simulink model "L4_MABX"  (R2018a)
settings: Solver=FixedStepDiscrete  StartTime=0.0  StopTime=Inf  FixedStep=0.01  RelTol=1e-3  EnableMultiTasking=on
PostLoadFcn:
  | , if any(exist('dsrtsu_mdlpostloadfcn', 'file') == [2, 3, 6]), try dsrtsu_mdlpostloadfcn('Execute', bdroot); catch fprintf('Error in PostLoadFcn (dsrtsu_mdlpostloadfcn) for model "%s":\n %s\n', bdroot, lasterr); end, end,
InitFcn:
  | disp([ptc_matlab_lib.isodatetime ' - ' bdroot(gcs) ' - Setting FixedStep to GLB_FIXED_STEP_SIZE_CPV']);
  | set_param(bdroot(gcs), 'FixedStep', num2str(GLB_FIXED_STEP_SIZE_CPV.Value));
undefined symbols (not defined in the file or in its folder): dsa_RTMapsManager, ENUM_CAN_STATUS_DIAG_T
libraries: PTC_MBDS_LIB x14, rtican x12, dsa_tcpip_lib x2, SUB_ECU_L4_MABX_HW_Interface_PIC_KW x2, rtiethxcplib x2, SUB_ECU_L4_MABX x1, simulink x1, rtmapslib x1
(part 2 of 2)

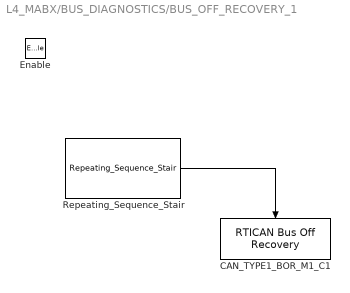
== system L4_MABX/BUS_DIAGNOSTICS/BUS_OFF_RECOVERY_1 ==
  Enable : EnablePort
      settings: AttributesFormatString=States when enabling: %<StatesWhenEnabling>
  CAN_TYPE1_BOR_M1_C1 : rtican/RTICAN Bus Off Recovery   Reserved1=[]  Reserved2=[]  Reserved3=[]  Reserved4=[]  SfcnRTICANBusOff=[]  DialogFcn=[]  BoardTypeNo=[]  BoardNo=[]  ChannelNo=[]  Parameters=[]  UnitName=[]  Revision=[]  UnitValues=[]  DSProperties=struct('RTI',struct('Version',uint32(3),'BlockType',struct('isSLSource',uint8(0),'isSLSink',uint8(1),'isHWSource',uint8(1),'isHWSink',uint8(0),'isSetup',uint8(0),'isInline',uint8(1),'isNonInline',uint8(0),'isInterrupt',uint8(0),'isChannelwise',uint8(0)),'IOBoardType','RTICAN','UnitType','NON_MESSAGE','Identifier','BUS_OFF_RECOVERY','DialogType','ML','BlockSet','RTICAN','SlaveProcessor','CAN'))  RTIBlockInterface=struct('DialogFcn','rtican_bus_off_recovery_gui','BlockDisplay',{{['\nCAN\n Bus Off Recovery'],'center'}},'TriggerPort',{{'either'}},'OutputPortsWidth',int32(0),'OutputPortsActive',0,'IconTransparency','on','InitLevel',3,'BlockName',struct('Token',{{'CAN_TYPE','_BOR_M','_C'}},'BlockParam',{{'BoardTypeNo','BoardNo','ChannelNo'}}))  RTIBlockParameters=struct('BoardTypeNo',{{1,'OFF',[]}},'BoardNo',{{1,'ON',[1 16]}},'ChannelNo',{{1,'ON',[1 2]}},'Parameters',{{struct('general',struct('isFromLib',0),'options',struct('TriggerType','either')),'OFF',[]}},'GroupId',{{struct('Group','RTICAN','No',1,'Behavior','NAMECHANGE','BlockType','SINK','NameChangeFlag',0),'OFF',[]}},'SFcnRTICANBusOff',{{0,'OFF',[]}},'TLCFileName',{{'rtican_bus_off_recovery','OFF',[]}})  RTISFcnParameters=struct('SFcnRTICANBusOff','struct','TLCFileName','char')  RTIBlockParaDefault=struct('BoardTypeNo',4302,'BoardNo',1,'ChannelNo',1,'Parameters',struct('general',struct('isFromLib',1),'options',struct('TriggerType','rising')),'GroupId',struct('Group',{{'RTICAN'}},'No',1,'Behavior',{{'NAMECHANGE'}},'BlockType',{{'SINK'}},'NameChangeFlag',0),'SFcnRTICANBusOff',0,'TLCFileName','rtican_bus_off_recovery')
      settings: AttributesFormatString=Group Id: RTICAN1\n  SourceProductName=dSPACE RTI CAN Blockset
  Repeating_Sequence_Stair : PTC_MBDS_LIB/Extras/Sources/Repeating_Sequence_Stair  OutValues=[true; false]  OutValues_prev=[true; false]  PTC_MBDS_BlockVersion=5.41  PTC_BlockType=PTC_MBDS_Repeating_Sequence_Stair
      settings: SourceProductName=PACCAR Technical Center MBDS Library
  wires:
  Repeating_Sequence_Stair/1 -> CAN_TYPE1_BOR_M1_C1/Trigger

== system L4_MABX/BUS_DIAGNOSTICS/BUS_OFF_RECOVERY_2 ==
  Enable : EnablePort
      settings: AttributesFormatString=States when enabling: %<StatesWhenEnabling>
  CAN_TYPE1_BOR_M1_C2 : rtican/RTICAN Bus Off Recovery   Reserved1=[]  Reserved2=[]  Reserved3=[]  Reserved4=[]  SfcnRTICANBusOff=[]  DialogFcn=[]  BoardTypeNo=[]  BoardNo=[]  ChannelNo=[]  Parameters=[]  UnitName=[]  Revision=[]  UnitValues=[]  DSProperties=struct('RTI',struct('Version',uint32(3),'BlockType',struct('isSLSource',uint8(0),'isSLSink',uint8(1),'isHWSource',uint8(1),'isHWSink',uint8(0),'isSetup',uint8(0),'isInline',uint8(1),'isNonInline',uint8(0),'isInterrupt',uint8(0),'isChannelwise',uint8(0)),'IOBoardType','RTICAN','UnitType','NON_MESSAGE','Identifier','BUS_OFF_RECOVERY','DialogType','ML','BlockSet','RTICAN','SlaveProcessor','CAN'))  RTIBlockInterface=struct('DialogFcn','rtican_bus_off_recovery_gui','BlockDisplay',{{['\nCAN\n Bus Off Recovery'],'center'}},'TriggerPort',{{'either'}},'OutputPortsWidth',int32(0),'OutputPortsActive',0,'IconTransparency','on','InitLevel',3,'BlockName',struct('Token',{{'CAN_TYPE','_BOR_M','_C'}},'BlockParam',{{'BoardTypeNo','BoardNo','ChannelNo'}}))  RTIBlockParameters=struct('BoardTypeNo',{{1,'OFF',[]}},'BoardNo',{{1,'ON',[1 16]}},'ChannelNo',{{2,'ON',[1 2]}},'Parameters',{{struct('general',struct('isFromLib',0),'options',struct('TriggerType','either')),'OFF',[]}},'GroupId',{{struct('Group','RTICAN','No',2,'Behavior','NAMECHANGE','BlockType','SINK','NameChangeFlag',0),'OFF',[]}},'SFcnRTICANBusOff',{{0,'OFF',[]}},'TLCFileName',{{'rtican_bus_off_recovery','OFF',[]}})  RTISFcnParameters=struct('SFcnRTICANBusOff','struct','TLCFileName','char')  RTIBlockParaDefault=struct('BoardTypeNo',4302,'BoardNo',1,'ChannelNo',1,'Parameters',struct('general',struct('isFromLib',1),'options',struct('TriggerType','rising')),'GroupId',struct('Group',{{'RTICAN'}},'No',1,'Behavior',{{'NAMECHANGE'}},'BlockType',{{'SINK'}},'NameChangeFlag',0),'SFcnRTICANBusOff',0,'TLCFileName','rtican_bus_off_recovery')
      settings: AttributesFormatString=Group Id: RTICAN2\n  SourceProductName=dSPACE RTI CAN Blockset
  Repeating_Sequence_Stair : PTC_MBDS_LIB/Extras/Sources/Repeating_Sequence_Stair  OutValues=[true; false]  OutValues_prev=[true; false]  PTC_MBDS_BlockVersion=5.41  PTC_BlockType=PTC_MBDS_Repeating_Sequence_Stair
      settings: SourceProductName=PACCAR Technical Center MBDS Library
  wires:
  Repeating_Sequence_Stair/1 -> CAN_TYPE1_BOR_M1_C2/Trigger

== system L4_MABX/BUS_DIAGNOSTICS/BUS_OFF_RECOVERY_3 ==
  Enable : EnablePort
      settings: AttributesFormatString=States when enabling: %<StatesWhenEnabling>
  CAN_TYPE1_BOR_M2_C1 : rtican/RTICAN Bus Off Recovery   Reserved1=[]  Reserved2=[]  Reserved3=[]  Reserved4=[]  SfcnRTICANBusOff=[]  DialogFcn=[]  BoardTypeNo=[]  BoardNo=[]  ChannelNo=[]  Parameters=[]  UnitName=[]  Revision=[]  UnitValues=[]  DSProperties=struct('RTI',struct('Version',uint32(3),'BlockType',struct('isSLSource',uint8(0),'isSLSink',uint8(1),'isHWSource',uint8(1),'isHWSink',uint8(0),'isSetup',uint8(0),'isInline',uint8(1),'isNonInline',uint8(0),'isInterrupt',uint8(0),'isChannelwise',uint8(0)),'IOBoardType','RTICAN','UnitType','NON_MESSAGE','Identifier','BUS_OFF_RECOVERY','DialogType','ML','BlockSet','RTICAN','SlaveProcessor','CAN'))  RTIBlockInterface=struct('DialogFcn','rtican_bus_off_recovery_gui','BlockDisplay',{{['\nCAN\n Bus Off Recovery'],'center'}},'TriggerPort',{{'either'}},'OutputPortsWidth',int32(0),'OutputPortsActive',0,'IconTransparency','on','InitLevel',3,'BlockName',struct('Token',{{'CAN_TYPE','_BOR_M','_C'}},'BlockParam',{{'BoardTypeNo','BoardNo','ChannelNo'}}))  RTIBlockParameters=struct('BoardTypeNo',{{1,'OFF',[]}},'BoardNo',{{2,'ON',[1 16]}},'ChannelNo',{{1,'ON',[1 2]}},'Parameters',{{struct('general',struct('isFromLib',0),'options',struct('TriggerType','either')),'OFF',[]}},'GroupId',{{struct('Group','RTICAN','No',3,'Behavior','NAMECHANGE','BlockType','SINK','NameChangeFlag',0),'OFF',[]}},'SFcnRTICANBusOff',{{0,'OFF',[]}},'TLCFileName',{{'rtican_bus_off_recovery','OFF',[]}})  RTISFcnParameters=struct('SFcnRTICANBusOff','struct','TLCFileName','char')  RTIBlockParaDefault=struct('BoardTypeNo',4302,'BoardNo',1,'ChannelNo',1,'Parameters',struct('general',struct('isFromLib',1),'options',struct('TriggerType','rising')),'GroupId',struct('Group',{{'RTICAN'}},'No',1,'Behavior',{{'NAMECHANGE'}},'BlockType',{{'SINK'}},'NameChangeFlag',0),'SFcnRTICANBusOff',0,'TLCFileName','rtican_bus_off_recovery')
      settings: AttributesFormatString=Group Id: RTICAN3\n  SourceProductName=dSPACE RTI CAN Blockset
  Repeating_Sequence_Stair : PTC_MBDS_LIB/Extras/Sources/Repeating_Sequence_Stair  OutValues=[true; false]  OutValues_prev=[true; false]  PTC_MBDS_BlockVersion=5.41  PTC_BlockType=PTC_MBDS_Repeating_Sequence_Stair
      settings: SourceProductName=PACCAR Technical Center MBDS Library
  wires:
  Repeating_Sequence_Stair/1 -> CAN_TYPE1_BOR_M2_C1/Trigger

== system L4_MABX/BUS_DIAGNOSTICS/BUS_OFF_RECOVERY_4 ==
  Enable : EnablePort
      settings: AttributesFormatString=States when enabling: %<StatesWhenEnabling>
  CAN_TYPE1_BOR_M2_C2 : rtican/RTICAN Bus Off Recovery   Reserved1=[]  Reserved2=[]  Reserved3=[]  Reserved4=[]  SfcnRTICANBusOff=[]  DialogFcn=[]  BoardTypeNo=[]  BoardNo=[]  ChannelNo=[]  Parameters=[]  UnitName=[]  Revision=[]  UnitValues=[]  DSProperties=struct('RTI',struct('Version',uint32(3),'BlockType',struct('isSLSource',uint8(0),'isSLSink',uint8(1),'isHWSource',uint8(1),'isHWSink',uint8(0),'isSetup',uint8(0),'isInline',uint8(1),'isNonInline',uint8(0),'isInterrupt',uint8(0),'isChannelwise',uint8(0)),'IOBoardType','RTICAN','UnitType','NON_MESSAGE','Identifier','BUS_OFF_RECOVERY','DialogType','ML','BlockSet','RTICAN','SlaveProcessor','CAN'))  RTIBlockInterface=struct('DialogFcn','rtican_bus_off_recovery_gui','BlockDisplay',{{['\nCAN\n Bus Off Recovery'],'center'}},'TriggerPort',{{'either'}},'OutputPortsWidth',int32(0),'OutputPortsActive',0,'IconTransparency','on','InitLevel',3,'BlockName',struct('Token',{{'CAN_TYPE','_BOR_M','_C'}},'BlockParam',{{'BoardTypeNo','BoardNo','ChannelNo'}}))  RTIBlockParameters=struct('BoardTypeNo',{{1,'OFF',[]}},'BoardNo',{{2,'ON',[1 16]}},'ChannelNo',{{2,'ON',[1 2]}},'Parameters',{{struct('general',struct('isFromLib',0),'options',struct('TriggerType','either')),'OFF',[]}},'GroupId',{{struct('Group','RTICAN','No',4,'Behavior','NAMECHANGE','BlockType','SINK','NameChangeFlag',0),'OFF',[]}},'SFcnRTICANBusOff',{{0,'OFF',[]}},'TLCFileName',{{'rtican_bus_off_recovery','OFF',[]}})  RTISFcnParameters=struct('SFcnRTICANBusOff','struct','TLCFileName','char')  RTIBlockParaDefault=struct('BoardTypeNo',4302,'BoardNo',1,'ChannelNo',1,'Parameters',struct('general',struct('isFromLib',1),'options',struct('TriggerType','rising')),'GroupId',struct('Group',{{'RTICAN'}},'No',1,'Behavior',{{'NAMECHANGE'}},'BlockType',{{'SINK'}},'NameChangeFlag',0),'SFcnRTICANBusOff',0,'TLCFileName','rtican_bus_off_recovery')
      settings: AttributesFormatString=Group Id: RTICAN4\n  SourceProductName=dSPACE RTI CAN Blockset
  Repeating_Sequence_Stair : PTC_MBDS_LIB/Extras/Sources/Repeating_Sequence_Stair  OutValues=[true; false]  OutValues_prev=[true; false]  PTC_MBDS_BlockVersion=5.41  PTC_BlockType=PTC_MBDS_Repeating_Sequence_Stair
      settings: SourceProductName=PACCAR Technical Center MBDS Library
  wires:
  Repeating_Sequence_Stair/1 -> CAN_TYPE1_BOR_M2_C2/Trigger

== system L4_MABX/BUS_DIAGNOSTICS/BUS_OFF_RECOVERY_5 ==
  Enable : EnablePort
      settings: AttributesFormatString=States when enabling: %<StatesWhenEnabling>
  CAN_TYPE1_BOR_M3_C1 : rtican/RTICAN Bus Off Recovery   Reserved1=[]  Reserved2=[]  Reserved3=[]  Reserved4=[]  SfcnRTICANBusOff=[]  DialogFcn=[]  BoardTypeNo=[]  BoardNo=[]  ChannelNo=[]  Parameters=[]  UnitName=[]  Revision=[]  UnitValues=[]  DSProperties=struct('RTI',struct('Version',uint32(3),'BlockType',struct('isSLSource',uint8(0),'isSLSink',uint8(1),'isHWSource',uint8(1),'isHWSink',uint8(0),'isSetup',uint8(0),'isInline',uint8(1),'isNonInline',uint8(0),'isInterrupt',uint8(0),'isChannelwise',uint8(0)),'IOBoardType','RTICAN','UnitType','NON_MESSAGE','Identifier','BUS_OFF_RECOVERY','DialogType','ML','BlockSet','RTICAN','SlaveProcessor','CAN'))  RTIBlockInterface=struct('DialogFcn','rtican_bus_off_recovery_gui','BlockDisplay',{{['\nCAN\n Bus Off Recovery'],'center'}},'TriggerPort',{{'either'}},'OutputPortsWidth',int32(0),'OutputPortsActive',0,'IconTransparency','on','InitLevel',3,'BlockName',struct('Token',{{'CAN_TYPE','_BOR_M','_C'}},'BlockParam',{{'BoardTypeNo','BoardNo','ChannelNo'}}))  RTIBlockParameters=struct('BoardTypeNo',{{1,'OFF',[]}},'BoardNo',{{3,'ON',[1 16]}},'ChannelNo',{{1,'ON',[1 2]}},'Parameters',{{struct('general',struct('isFromLib',0),'options',struct('TriggerType','either')),'OFF',[]}},'GroupId',{{struct('Group','RTICAN','No',5,'Behavior','NAMECHANGE','BlockType','SINK','NameChangeFlag',0),'OFF',[]}},'SFcnRTICANBusOff',{{0,'OFF',[]}},'TLCFileName',{{'rtican_bus_off_recovery','OFF',[]}})  RTISFcnParameters=struct('SFcnRTICANBusOff','struct','TLCFileName','char')  RTIBlockParaDefault=struct('BoardTypeNo',4302,'BoardNo',1,'ChannelNo',1,'Parameters',struct('general',struct('isFromLib',1),'options',struct('TriggerType','rising')),'GroupId',struct('Group',{{'RTICAN'}},'No',1,'Behavior',{{'NAMECHANGE'}},'BlockType',{{'SINK'}},'NameChangeFlag',0),'SFcnRTICANBusOff',0,'TLCFileName','rtican_bus_off_recovery')
      settings: AttributesFormatString=Group Id: RTICAN5\n  SourceProductName=dSPACE RTI CAN Blockset
  Repeating_Sequence_Stair : PTC_MBDS_LIB/Extras/Sources/Repeating_Sequence_Stair  OutValues=[true; false]  OutValues_prev=[true; false]  PTC_MBDS_BlockVersion=5.41  PTC_BlockType=PTC_MBDS_Repeating_Sequence_Stair
      settings: SourceProductName=PACCAR Technical Center MBDS Library
  wires:
  Repeating_Sequence_Stair/1 -> CAN_TYPE1_BOR_M3_C1/Trigger

== system L4_MABX/BUS_DIAGNOSTICS/BUS_OFF_RECOVERY_6 ==
  Enable : EnablePort
      settings: AttributesFormatString=States when enabling: %<StatesWhenEnabling>
  CAN_TYPE1_BOR_M3_C2 : rtican/RTICAN Bus Off Recovery   Reserved1=[]  Reserved2=[]  Reserved3=[]  Reserved4=[]  SfcnRTICANBusOff=[]  DialogFcn=[]  BoardTypeNo=[]  BoardNo=[]  ChannelNo=[]  Parameters=[]  UnitName=[]  Revision=[]  UnitValues=[]  DSProperties=struct('RTI',struct('Version',uint32(3),'BlockType',struct('isSLSource',uint8(0),'isSLSink',uint8(1),'isHWSource',uint8(1),'isHWSink',uint8(0),'isSetup',uint8(0),'isInline',uint8(1),'isNonInline',uint8(0),'isInterrupt',uint8(0),'isChannelwise',uint8(0)),'IOBoardType','RTICAN','UnitType','NON_MESSAGE','Identifier','BUS_OFF_RECOVERY','DialogType','ML','BlockSet','RTICAN','SlaveProcessor','CAN'))  RTIBlockInterface=struct('DialogFcn','rtican_bus_off_recovery_gui','BlockDisplay',{{['\nCAN\n Bus Off Recovery'],'center'}},'TriggerPort',{{'either'}},'OutputPortsWidth',int32(0),'OutputPortsActive',0,'IconTransparency','on','InitLevel',3,'BlockName',struct('Token',{{'CAN_TYPE','_BOR_M','_C'}},'BlockParam',{{'BoardTypeNo','BoardNo','ChannelNo'}}))  RTIBlockParameters=struct('BoardTypeNo',{{1,'OFF',[]}},'BoardNo',{{3,'ON',[1 16]}},'ChannelNo',{{2,'ON',[1 2]}},'Parameters',{{struct('general',struct('isFromLib',0),'options',struct('TriggerType','either')),'OFF',[]}},'GroupId',{{struct('Group','RTICAN','No',6,'Behavior','NAMECHANGE','BlockType','SINK','NameChangeFlag',0),'OFF',[]}},'SFcnRTICANBusOff',{{0,'OFF',[]}},'TLCFileName',{{'rtican_bus_off_recovery','OFF',[]}})  RTISFcnParameters=struct('SFcnRTICANBusOff','struct','TLCFileName','char')  RTIBlockParaDefault=struct('BoardTypeNo',4302,'BoardNo',1,'ChannelNo',1,'Parameters',struct('general',struct('isFromLib',1),'options',struct('TriggerType','rising')),'GroupId',struct('Group',{{'RTICAN'}},'No',1,'Behavior',{{'NAMECHANGE'}},'BlockType',{{'SINK'}},'NameChangeFlag',0),'SFcnRTICANBusOff',0,'TLCFileName','rtican_bus_off_recovery')
      settings: AttributesFormatString=Group Id: RTICAN6\n  SourceProductName=dSPACE RTI CAN Blockset
  Repeating_Sequence_Stair : PTC_MBDS_LIB/Extras/Sources/Repeating_Sequence_Stair  OutValues=[true; false]  OutValues_prev=[true; false]  PTC_MBDS_BlockVersion=5.41  PTC_BlockType=PTC_MBDS_Repeating_Sequence_Stair
      settings: SourceProductName=PACCAR Technical Center MBDS Library
  wires:
  Repeating_Sequence_Stair/1 -> CAN_TYPE1_BOR_M3_C2/Trigger

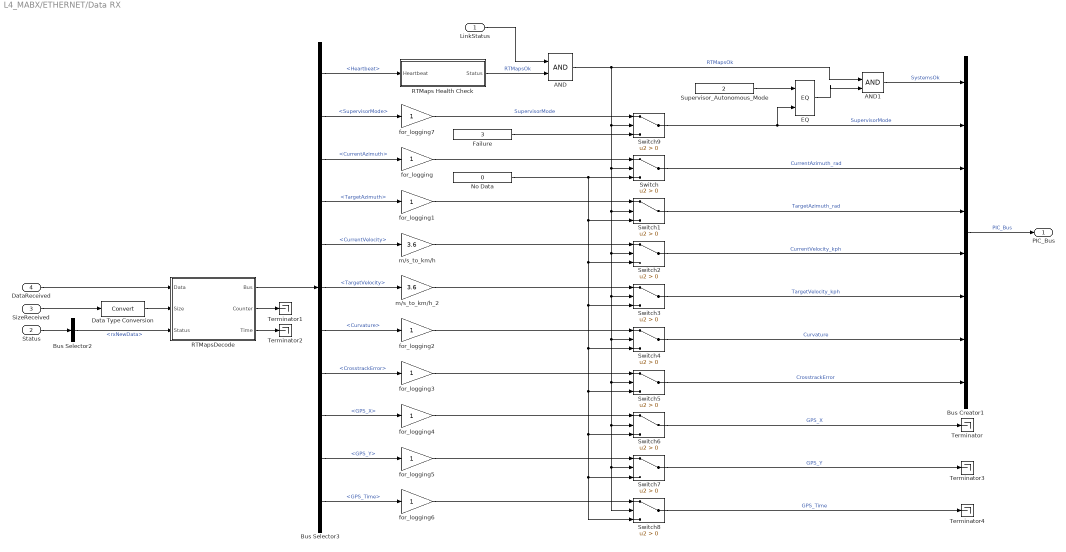
== system L4_MABX/ETHERNET/Data RX ==
  LinkStatus : Inport
  Status : Inport  Port=2
  SizeReceived : Inport  Port=3
  DataReceived : Inport  Port=4
  AND : Logic  IconShape=distinctive  AllPortsSameDT=off  OutDataTypeStr=boolean
  AND1 : Logic  IconShape=distinctive  AllPortsSameDT=off  OutDataTypeStr=boolean
  Bus Creator1 : BusCreator  Inputs=8
  Bus Selector2 : BusSelector  OutputSignals=rxNewData
  Bus Selector3 : BusSelector  OutputSignals=Heartbeat,SupervisorMode,CurrentAzimuth,TargetAzimuth,CurrentVelocity,TargetVelocity,Curvature,CrosstrackError,GPS_X,GPS_Y,GPS_Time
  Data Type Conversion : DataTypeConversion
  EQ : PTC_MBDS_LIB/MBDS Standard Library/Basic Operations/Logic and Bit Operations/EQ  InputSameDT=on  PTC_MBDS_BlockVersion=5.41  PTC_BlockType=PTC_MBDS_EQ
      settings: SourceProductName=PACCAR Technical Center MBDS Library
  Failure : Constant  Value=3  OutDataTypeStr=uint8
  No Data : Constant  Value=0  OutDataTypeStr=double
  RTMaps Health Check : Subsystem
  RTMapsDecode : Subsystem  AncestorBlock=rtmapslib/RTMapsDecode  InitFcn=dsa_RTMapsManager.ContainsImplementation(gcb);  mask(dsa_RTMaps_Receive){paramBusName=RTMapsRX}
      settings: AttributesFormatString=Bus: %<paramBusName>  OpenFcn=dsa_RTMaps_rx_gui(gcbh);
      mask DialogControl textField Prompt: Bus Name:
  Supervisor_Autonomous_Mode : Constant  Value=2  OutDataTypeStr=Inherit: Inherit via back propagation
  Switch{,1..9} (10 alike) : Switch  Criteria=u2 > Threshold
  Terminator{,1..4} (5 alike) : Terminator
  for_logging{,1..6} (7 alike) : Gain
  for_logging7 : Gain  OutDataTypeStr=int8
  m/s_to_km/h : Gain  Gain=3.6
  m/s_to_km/h_2 : Gain  Gain=3.6
  PIC_Bus : Outport
  wires:
  Failure/1 -> Switch9/3
  Switch7/1 -> Terminator3/1  "GPS_Y"
  Switch2/1 -> Bus Creator1/5  "CurrentVelocity_kph"
  for_logging5/1 -> Switch7/1
  for_logging7/1 -> Switch9/1  "SupervisorMode"
  m/s_to_km/h_2/1 -> Switch3/1
  Switch8/1 -> Terminator4/1  "GPS_Time"
  LinkStatus/1 -> AND/1
  for_logging3/1 -> Switch5/1
  for_logging4/1 -> Switch6/1
  Switch5/1 -> Bus Creator1/8  "CrosstrackError"
  No Data/1 -> Switch/3, Switch1/3, Switch2/3, Switch3/3, Switch5/3, Switch6/3, Switch7/3, Switch8/3, Switch4/3
  Switch1/1 -> Bus Creator1/4  "TargetAzimuth_rad"
  m/s_to_km/h/1 -> Switch2/1
  Bus Selector3/10 -> for_logging5/1  "<GPS_Y>"
  Bus Selector3/11 -> for_logging6/1  "<GPS_Time>"
  Bus Selector3/8 -> for_logging3/1  "<CrosstrackError>"
  Bus Selector3/5 -> m/s_to_km/h/1  "<CurrentVelocity>"
  Switch6/1 -> Terminator/1  "GPS_X"
  RTMapsDecode/1(Bus) -> Bus Selector3/1
  Data Type Conversion/1 -> RTMapsDecode/2(Size)
  Bus Creator1/1 -> PIC_Bus/1  "PIC_Bus"
  Switch4/1 -> Bus Creator1/7  "Curvature"
  Bus Selector3/3 -> for_logging/1  "<CurrentAzimuth>"
  RTMapsDecode/2(Counter) -> Terminator1/1
  Bus Selector3/6 -> m/s_to_km/h_2/1  "<TargetVelocity>"
  for_logging1/1 -> Switch1/1
  RTMapsDecode/3(Time) -> Terminator2/1
  for_logging6/1 -> Switch8/1
  Bus Selector3/9 -> for_logging4/1  "<GPS_X>"
  Bus Selector3/7 -> for_logging2/1  "<Curvature>"
  Bus Selector3/1 -> RTMaps Health Check/1(Heartbeat)  "<Heartbeat>"
  Switch3/1 -> Bus Creator1/6  "TargetVelocity_kph"
  for_logging/1 -> Switch/1
  Bus Selector3/4 -> for_logging1/1  "<TargetAzimuth>"
  AND/1 -> AND1/1, Switch9/2, Switch8/2, Switch7/2, Switch6/2, Switch5/2, Switch4/2, Switch3/2, Switch2/2, Switch1/2, Switch/2  "RTMapsOk"
  RTMaps Health Check/1(Status) -> AND/2  "RTMapsOk"
  Bus Selector3/2 -> for_logging7/1  "<SupervisorMode>"
  Bus Selector2/1 -> RTMapsDecode/3(Status)  "<rxNewData>"
  for_logging2/1 -> Switch4/1
  Switch/1 -> Bus Creator1/3  "CurrentAzimuth_rad"
  Switch9/1 -> Bus Creator1/2, EQ/2  "SupervisorMode"
  Status/1 -> Bus Selector2/1
  DataReceived/1 -> RTMapsDecode/1(Data)
  SizeReceived/1 -> Data Type Conversion/1
  Supervisor_Autonomous_Mode/1 -> EQ/1
  AND1/1 -> Bus Creator1/1  "SystemsOk"
  EQ/1 -> AND1/2

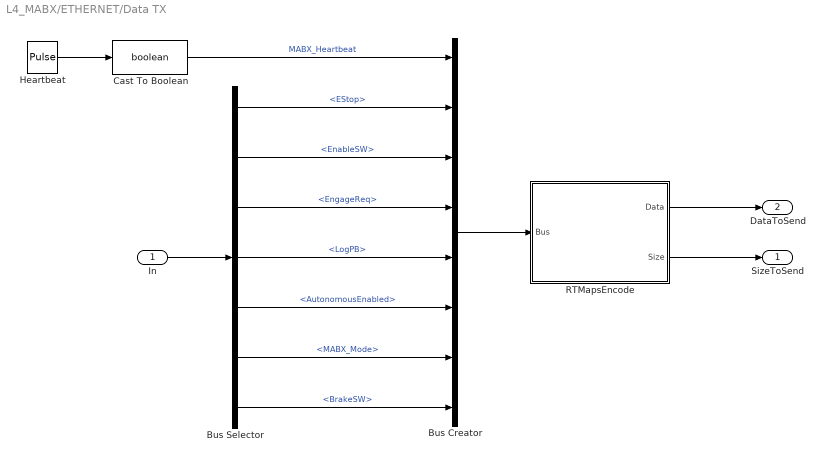
== system L4_MABX/ETHERNET/Data TX ==
  In : Inport
  Bus Creator : BusCreator  Inputs=8  OutDataTypeStr=Bus: RTMapsTX  NonVirtualBus=on
  Bus Selector : BusSelector  OutputSignals=INPUTS.DIO_Bus.EStop,INPUTS.DIO_Bus.EnableSW,10msTask.AutonomousState.EngageReq,INPUTS.DIO_Bus.LogPB,10msTask.AutonomousState.AutonomousEnabled,10msTask.AutonomousState.MABX_Mode,INPUTS.DIO_Bus.BrakeSW
  Cast To Boolean : DataTypeConversion  OutDataTypeStr=boolean
  Heartbeat : DiscretePulseGenerator  Period=10  PulseWidth=5  SampleTime=0.01
  RTMapsEncode : Subsystem  AncestorBlock=rtmapslib/RTMapsEncode  InitFcn=dsa_RTMapsManager.ContainsImplementation(gcb);  mask(dsa_RTMaps_Transmit){TimestampMode=Simulation Time}
      mask prompts: TimestampMode "Time source:"
      mask Help: eval('dsa_RTMapsManager.Documentation(''RTMaps Encode Block'');');
      mask TypeOptions TimestampMode: Simulation Time | Real Time
      mask DialogControl Control3 Prompt: This parameter is only evaluated if the target platform is a Microautobox. Otherwise, it will be ignored.
      mask DialogControl Control2 Prompt: Depending on your selection, this block will either transmit the current Simulation or the current Real Time to RTMaps.
  SizeToSend : Outport
  DataToSend : Outport  Port=2
  wires:
  Bus Selector/3 -> Bus Creator/4  "<EngageReq>"
  Bus Selector/1 -> Bus Creator/2  "<EStop>"
  Bus Selector/2 -> Bus Creator/3  "<EnableSW>"
  Bus Selector/6 -> Bus Creator/7  "<MABX_Mode>"
  Bus Selector/5 -> Bus Creator/6  "<AutonomousEnabled>"
  In/1 -> Bus Selector/1
  Heartbeat/1 -> Cast To Boolean/1
  Cast To Boolean/1 -> Bus Creator/1  "MABX_Heartbeat"
  Bus Creator/1 -> RTMapsEncode/1(Bus)
  RTMapsEncode/1(Data) -> DataToSend/1
  RTMapsEncode/2(Size) -> SizeToSend/1
  Bus Selector/4 -> Bus Creator/5  "<LogPB>"
  Bus Selector/7 -> Bus Creator/8  "<BrakeSW>"

== system L4_MABX/RTI Data/RTI Data Store ==
  RTI Data Store : Subsystem  mask(RTI_DATA_STORE){}
      mask help:
      | RTI Data Store Block. This block is used by RTI to store internal model dependent data. Deleting this block will result in data loss.
      |
      | NEVER DELETE, COPY, OR MODIFY THIS BLOCK!
      mask Help:
      | RTI Data Store Block. This block is used by RTI to store internal model dependent data. Deleting this block will result in data loss.
      | 
      | NEVER DELETE, COPY, OR MODIFY THIS BLOCK!
      mask Display: text(0.5, 0.5, ' ', 'HorizontalAlignment', 'center');

== system L4_MABX/VersionInformation/EnabledSubsystem ==
  Enable : EnablePort
      settings: AttributesFormatString=States when enabling: %<StatesWhenEnabling>
  Constant : PTC_MBDS_LIB/Extras/Sources/Constant  Value2=GLB_SWVERSION_CPV  PTC_MBDS_BlockVersion=5.41  PTC_BlockType=PTC_MBDS_Constant
      settings: SourceProductName=PACCAR Technical Center MBDS Library
      settings: AttributesFormatString=|
      | Value: <1 X 100>
      | Unit: 'ASCII'
  Terminator : Terminator
      settings: InitFcn=|
      | try
      |    MBDS_BlockCallback('Update', gcb);
      | end
  wires:
  Constant/1 -> Terminator/1  "GLB_SWVERSION_CPV_"

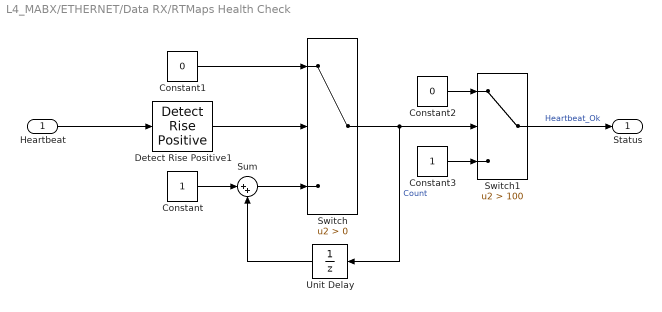
== system L4_MABX/ETHERNET/Data RX/RTMaps Health Check ==
  Heartbeat : Inport
  Constant : Constant
  Constant1 : Constant  Value=0
  Constant2 : Constant  Value=0  OutDataTypeStr=boolean
  Constant3 : Constant  OutDataTypeStr=boolean
  Detect Rise Positive1 : simulink/Logic and Bit Operations/Detect Rise Positive  vinit=0  OutDataTypeStr=boolean
  Sum : Sum  Inputs=|++
  Switch : Switch  Criteria=u2 > Threshold
  Switch1 : Switch  Criteria=u2 > Threshold  Threshold=100
  Unit Delay : UnitDelay  SampleTime=-1
  Status : Outport
  wires:
  Switch1/1 -> Status/1  "Heartbeat_Ok"
  Constant3/1 -> Switch1/3
  Detect Rise Positive1/1 -> Switch/2
  Constant1/1 -> Switch/1
  Switch/1 -> Unit Delay/1, Switch1/2  "Count"
  Heartbeat/1 -> Detect Rise Positive1/1
  Sum/1 -> Switch/3
  Constant2/1 -> Switch1/1
  Constant/1 -> Sum/1
  Unit Delay/1 -> Sum/2

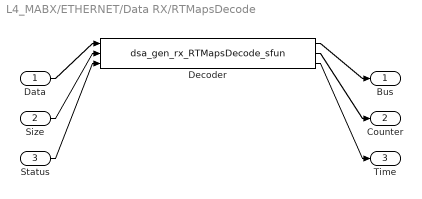
== system L4_MABX/ETHERNET/Data RX/RTMapsDecode ==
  Data : Inport
  Size : Inport  Port=2
  Status : Inport  Port=3
  Decoder : S-Function  FunctionName=dsa_gen_rx_RTMapsDecode_sfun  SFunctionDeploymentMode=off  EnableBusSupport=off  mask(Legacy Function){SFunctionSpec=void Update_Rx_RTMapsDecode(uint8 u1[], uint32 u2, uint32 u3, RTMapsRX y1[1], int32 y2[1], double y3[1]), ShowSpec=on}
      mask prompts: ShowSpec "Display function specification"
      mask help:
      | This block allows you to call the legacy functions specified by the following Legacy Code Tool definition:
      | def.SFunctionName = 'dsa_gen_rx_RTMapsDecode_sfun';
      | def.OutputFcnSpec = 'void Update_Rx_RTMapsDecode(uint8 u1[], uint32 u2, uint32 u3, RTMapsRX y1[1], int32 y2[1], double y3[1])';
      | def.StartFcnSpec = 'void Init_Rx_RTMapsDecode()';
      | def.HeaderFiles = {'dsa_gen_rx_RTMapsDecode.h'};
      | def.SourceFiles = {'dsa_gen_rx_RTMapsDecode.c'};
      mask Help: <p>This block was generated automatically by the Legacy Code Tool. For detailed help on this tool, call<a href="matlab:legacy_code('help')"> legacy_code('help')</a>.</p>
      mask Callback ShowSpec:
      | if strcmp(get_param(gcbh, 'ShowSpec'), 'on')
      |   set_param(gcbh, 'MaskDisplay', sprintf('fprintf(''%s'');', get_param(gcbh, 'SFunctionSpec')));
      | else
      |   set_param(gcbh, 'MaskDisplay', sprintf('fprintf(''%s'');', get_param(gcbh, 'FunctionName')));
      | end
      mask Display: fprintf('void Update_Rx_RTMapsDecode(uint8 u1[], uint32 u2, uint32 u3, RTMapsRX y1[1], int32 y2[1], double y3[1])');
  Bus : Outport
  Counter : Outport  Port=2
  Time : Outport  Port=3
  wires:
  Data/1 -> Decoder/1
  Size/1 -> Decoder/2
  Status/1 -> Decoder/3
  Decoder/1 -> Bus/1
  Decoder/2 -> Counter/1
  Decoder/3 -> Time/1

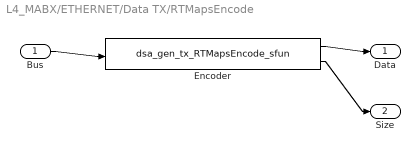
== system L4_MABX/ETHERNET/Data TX/RTMapsEncode ==
  Bus : Inport
  Encoder : S-Function  FunctionName=dsa_gen_tx_RTMapsEncode_sfun  SFunctionDeploymentMode=off  EnableBusSupport=off  mask(Legacy Function){SFunctionSpec=void Update_Tx_RTMapsEncode(RTMapsTX u1[1], uint8 y1[24], uint32 y2[1]), ShowSpec=on}
      mask prompts: ShowSpec "Display function specification"
      mask help:
      | This block allows you to call the legacy functions specified by the following Legacy Code Tool definition:
      | def.SFunctionName = 'dsa_gen_tx_RTMapsEncode_sfun';
      | def.OutputFcnSpec = 'void Update_Tx_RTMapsEncode(RTMapsTX u1[1], uint8 y1[24], uint32 y2[1])';
      | def.StartFcnSpec = 'void Init_Tx_RTMapsEncode()';
      | def.HeaderFiles = {'dsa_gen_tx_RTMapsEncode.h'};
      mask Help: <p>This block was generated automatically by the Legacy Code Tool. For detailed help on this tool, call<a href="matlab:legacy_code('help')"> legacy_code('help')</a>.</p>
      mask Callback ShowSpec:
      | if strcmp(get_param(gcbh, 'ShowSpec'), 'on')
      |   set_param(gcbh, 'MaskDisplay', sprintf('fprintf(''%s'');', get_param(gcbh, 'SFunctionSpec')));
      | else
      |   set_param(gcbh, 'MaskDisplay', sprintf('fprintf(''%s'');', get_param(gcbh, 'FunctionName')));
      | end
      mask Display: fprintf('void Update_Tx_RTMapsEncode(RTMapsTX u1[1], uint8 y1[24], uint32 y2[1])');
  Data : Outport
  Size : Outport  Port=2
  wires:
  Bus/1 -> Encoder/1
  Encoder/1 -> Data/1
  Encoder/2 -> Size/1

== system L4_MABX/RTI Data/RTI Data Store/RTI Data Store ==
  RTI Data Store : Subsystem  mask(RTI_DATA_STORE){}
      mask help:
      | RTI Data Store Block. This block is used by RTI to store internal model dependent data. Deleting this block will result in data loss.
      |
      | NEVER DELETE, COPY, OR MODIFY THIS BLOCK!
      mask Help:
      | RTI Data Store Block. This block is used by RTI to store internal model dependent data. Deleting this block will result in data loss.
      | 
      | NEVER DELETE, COPY, OR MODIFY THIS BLOCK!
      mask Display: text(0.5, 0.5, ' ', 'HorizontalAlignment', 'center');

== system L4_MABX/RTI Data/RTI Data Store/RTI Data Store/RTI Data Store ==
  RTI Data Store : Subsystem  mask(RTI_DATA_STORE){}
      mask help:
      | RTI Data Store Block. This block is used by RTI to store internal model dependent data. Deleting this block will result in data loss.
      |
      | NEVER DELETE, COPY, OR MODIFY THIS BLOCK!
      mask Help:
      | RTI Data Store Block. This block is used by RTI to store internal model dependent data. Deleting this block will result in data loss.
      | 
      | NEVER DELETE, COPY, OR MODIFY THIS BLOCK!
      mask Display: text(0.5, 0.5, ' ', 'HorizontalAlignment', 'center');

== system L4_MABX/RTI Data/RTI Data Store/RTI Data Store/RTI Data Store/RTI Data Store ==
